simulink model "fourth1"  (R2021b)
settings: Solver=VariableStepAuto  StartTime=0.0  StopTime=30  RelTol=1e-3
settings Model: Creator=minna  LastModifiedBy=minna

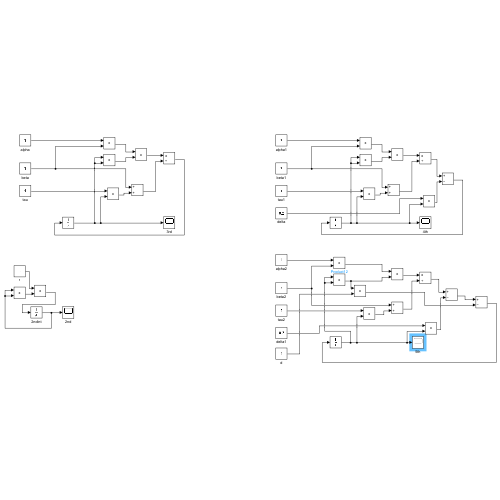
[thumbnail: Simulink's stored preview of the top-level diagram]
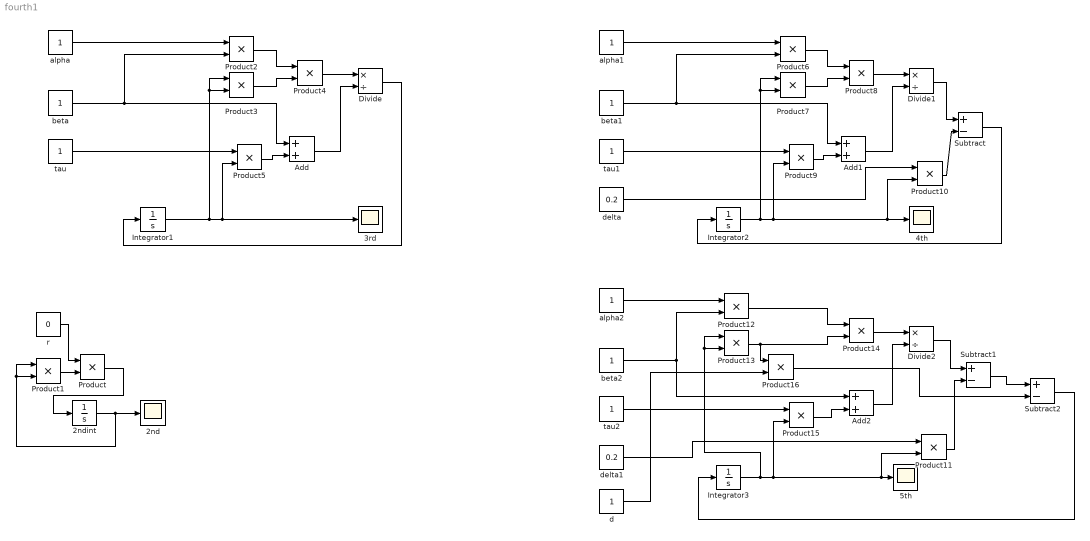
== system fourth1 ==
  2nd : Scope
  2ndint : Integrator  InitialCondition=2
  3rd : Scope
  4th : Scope
  5th : Scope
  Add : Sum
  Add1 : Sum
  Add2 : Sum
  Divide : Product  Inputs=*/
  Divide1 : Product  Inputs=*/
  Divide2 : Product  Inputs=*/
  Integrator1 : Integrator  InitialCondition=2
  Integrator2 : Integrator  InitialCondition=2
  Integrator3 : Integrator  InitialCondition=2
  Product{,1..16} (17 alike) : Product
  Subtract : Sum  Inputs=+-
  Subtract1 : Sum  Inputs=+-
  Subtract2 : Sum  Inputs=+-
  alpha : Constant
  alpha1 : Constant
  alpha2 : Constant
  beta : Constant
  beta1 : Constant
  beta2 : Constant
  d : Constant
  delta : Constant  Value=0.2
  delta1 : Constant  Value=0.2
  r : Constant  Value=0
  tau : Constant
  tau1 : Constant
  tau2 : Constant
  wires:
  r/1 -> Product/1
  2ndint/1 -> 2nd/1, Product1/1, Product1/2
  Product1/1 -> Product/2
  Product/1 -> 2ndint/1
  alpha/1 -> Product2/1
  beta/1 -> Add/1, Product2/2
  Integrator1/1 -> Product5/2, 3rd/1, Product3/1, Product3/2
  Product3/1 -> Product4/2
  Product2/1 -> Product4/1
  Product4/1 -> Divide/1
  tau/1 -> Product5/1
  Product5/1 -> Add/2
  Add/1 -> Divide/2
  Divide/1 -> Integrator1/1
  tau1/1 -> Product9/1
  Product9/1 -> Add1/2
  Integrator2/1 -> 4th/1, Product10/2, Product9/2, Product7/1, Product7/2
  Product6/1 -> Product8/1
  beta1/1 -> Add1/1, Product6/2
  Product7/1 -> Product8/2
  alpha1/1 -> Product6/1
  Product8/1 -> Divide1/1
  Add1/1 -> Divide1/2
  delta/1 -> Product10/1
  Divide1/1 -> Subtract/1
  Product10/1 -> Subtract/2
  Subtract/1 -> Integrator2/1
  Add2/1 -> Divide2/2
  Product14/1 -> Divide2/1
  Product13/1 -> Product16/1, Product14/2
  beta2/1 -> Add2/1, Product12/2
  Product15/1 -> Add2/2
  tau2/1 -> Product15/1
  Product12/1 -> Product14/1
  Integrator3/1 -> Product11/2, 5th/1, Product15/2, Product13/1, Product13/2
  Product11/1 -> Subtract1/2
  Divide2/1 -> Subtract1/1
  Subtract1/1 -> Subtract2/1
  delta1/1 -> Product11/1
  alpha2/1 -> Product12/1
  d/1 -> Product16/2
  Product16/1 -> Subtract2/2
  Subtract2/1 -> Integrator3/1
